simulink model "Trab_Tulior"  (R2020a)
settings: Solver=ode45  StartTime=0.0  StopTime=10  RelTol=1e-3  EnableMultiTasking=on
libraries: simulink x2
settings Model: Creator=20211en20246  LastModifiedBy=João Fernando Rangel
settings DataIOCC: LimitDataPoints=on  SaveFormat=Array  ReturnWorkspaceOutputs=off
settings OptimizationCC: LifeSpan=inf
settings DebuggingCC: UnderspecifiedInitializationDetection=Classic  MergeDetectMultiDrivingBlocksExec=none  SolverPrmCheckMsg=warning  SFUnexpectedBacktrackingDiag=warning  SFNoUnconditionalDefaultTransitionDiag=warning  SFExecutionAtInitializationDiag=none  ArithmeticOperatorsInVariantConditions=warning
settings HardwareCC: ProdBitPerPointer=32  ProdBitPerSizeT=32  ProdBitPerPtrDiffT=32  ProdLargestAtomicFloat=None  ProdIntDivRoundTo=Undefined  ProdEndianess=Unspecified  ProdWordSize=32  ProdHWDeviceType=32-bit Generic
settings ModelReferenceCC: PropagateSignalLabelsOutOfModel=off
settings SFSimCC: SimUseLocalCustomCode=off  CustomCodeUndefinedFunction=UseInterfaceOnly
settings RTWCC: RTWUseLocalCustomCode=off
settings CodeAppCC: StateflowObjectComments=on
settings GRTTargetCC: TargetLangStandard=C89/C90 (ANSI)
settings ConfigComp: CovMetricSettings=dw  CovHtmlReporting=on  CovSaveCumulativeToWorkspaceVar=on  CovSaveSingleToWorkspaceVar=on  CovExternalEMLEnable=off

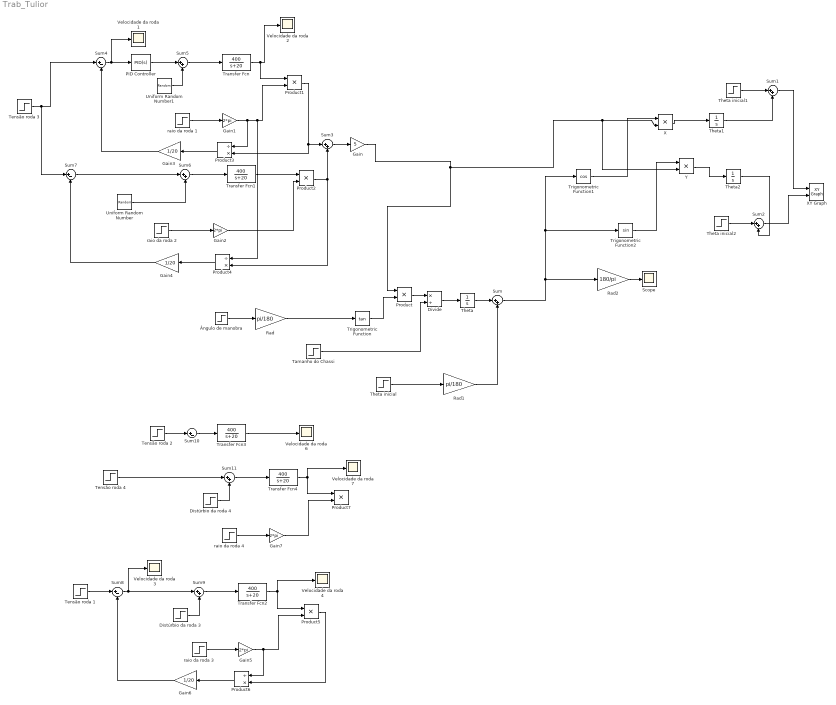
== system Trab_Tulior ==
  Distúrbio da roda 3 : Step  Time=0  After=0  SampleTime=0
  Distúrbio da roda 4 : Step  Time=0  After=0  SampleTime=0
  Divide : Product  Inputs=*/
  Gain : Gain  Gain=5
  Gain{1..2,5,7} (4 alike) : Gain  Gain=2*pi
  Gain3 : Gain  Gain=1/20
  Gain4 : Gain  Gain=1/20
  Gain6 : Gain  Gain=1/20
  PID Controller : simulink/Continuous/PID Controller  Controller=PID  Form=Parallel  TimeDomain=Continuous-time  UseExternalTs=off  SampleTime=-1  IntegratorMethod=Forward Euler  FilterMethod=Forward Euler  ControllerParametersSource=internal  P=77.31  I=171.77  D=1.28  UseFilter=on  N=100  TunerSelectOption=Transfer Function Based (PID Tuner App)  InitialConditionSource=internal  InitialConditionForIntegrator=0  InitialConditionForFilter=0  DifferentiatorICPrevScaledInput=0  ExternalReset=none  TrackingMode=off  Kt=1  LimitOutput=off  UpperSaturationLimit=inf  LowerSaturationLimit=-inf  LinearizeAsGain=on  AntiWindupMode=none  Kb=1  POutMin=[]  POutMax=[]  IOutMin=[]  IOutMax=[]  DOutMin=[]  DOutMax=[]  NOutMin=[]  NOutMax=[]  SumOutMin=[]  SumOutMax=[]  SaturationOutMin=[]  SaturationOutMax=[]  PParamMin=[]  PParamMax=[]  IParamMin=[]  IParamMax=[]  DParamMin=[]  DParamMax=[]  NParamMin=[]  NParamMax=[]  KbParamMin=[]  KbParamMax=[]  KtParamMin=[]  KtParamMax=[]  KbOutMin=[]  KbOutMax=[]  KtOutMin=[]  KtOutMax=[]  IntegratorOutMin=[]  IntegratorOutMax=[]  FilterOutMin=[]  FilterOutMax=[]  SumI1OutMin=[]  SumI1OutMax=[]  SumI2OutMin=[]  SumI2OutMax=[]  SumI3OutMin=[]  SumI3OutMax=[]  SumI4OutMin=[]  SumI4OutMax=[]  SumDOutMin=[]  SumDOutMax=[]  DifferentiatorOutMin=[]  DifferentiatorOutMax=[]  FilterDiffOutCoefMin=[]  FilterDiffOutCoefMax=[]  ReciprocalOutMin=[]  ReciprocalOutMax=[]  SumDenOutMin=[]  SumDenOutMax=[]  SumNumOutMin=[]  SumNumOutMax=[]  DivideOutMin=[]  DivideOutMax=[]  UdiffTsProdOutMin=[]  UdiffTsProdOutMax=[]  NTsProdOutMin=[]  NTsProdOutMax=[]  UintegralTsProdOutMin=[]  UintegralTsProdOutMax=[]  UngainTsProdOutMin=[]  UngainTsProdOutMax=[]  IntegratorContinuousStateAttributes=''  IntegratorStateMustResolveToSignalObject=off  IntegratorRTWStateStorageClass=Auto  FilterContinuousStateAttributes=''  FilterStateMustResolveToSignalObject=off  FilterRTWStateStorageClass=Auto  ParallelPVariant=InternalParameters  IdealPVariant=Disabled  IVariant=InternalParameters  DVariant=InternalParameters  IntegratorVariant=Continuous  SatVariant=Disabled  AWVariant=Passthrough  PCopyVariant=Disabled  TRVariant=Disabled  FdbkBlocksVariant=Forward  IdealPFdbkVariant=Disabled  SatFdbkVariant=Disabled  DerivativeFilterVariant=ContFilter  NVariant=InternalParameters  NCopyVariant=Disabled  FilterICVariant=InternalICsFilter  IntegratorICVariant=InternalICs  ExternalResetVariant=Disabled  TRSumVariant=Passthrough  SumFdbkVariant=Disabled  SumVariant=Sum_PID  TsampFilterVariant=InternalTs  TsampNgainVariant=Passthrough  TsampIntegralVariant=Passthrough
  Product{,1..2,5,7} (5 alike) : Product
  Product3 : Product  Inputs=/*
  Product4 : Product  Inputs=/*
  Product6 : Product  Inputs=/*
  Rad : Gain  Gain=pi/180
  Rad1 : Gain  Gain=pi/180
  Rad2 : Gain  Gain=180/pi
  Scope : Scope
  Sum{,1..3,5..6,9,11} (8 alike) : Sum  Inputs=|++
  Sum{4,7..8,10} (4 alike) : Sum  Inputs=|+-
  Tamanho do Chassi : Step  Time=0  After=0.44  SampleTime=0
  Tensão roda 1 : Step  Time=0  SampleTime=0
  Tensão roda 2 : Step  SampleTime=0
  Tensão roda 3 : Step  Time=0  SampleTime=0
  Tensão roda 4 : Step  Time=0  SampleTime=0
  Theta : Integrator
  Theta inicial : Step  Time=0  After=0  SampleTime=0
  Theta inicial1 : Step  Time=0  After=0  SampleTime=0
  Theta inicial2 : Step  Time=0  After=0  SampleTime=0
  Theta1 : Integrator
  Theta2 : Integrator
  Transfer Fcn{,1..4} (5 alike) : TransferFcn  Numerator=[400]  Denominator=[1 20]
  Trigonometric Function : Trigonometry  Operator=tan
  Trigonometric Function1 : Trigonometry  Operator=cos
  Trigonometric Function2 : Trigonometry
  Uniform Random Number : UniformRandomNumber  Minimum=-0.1  Maximum=5  SampleTime=0.1
  Uniform Random Number1 : UniformRandomNumber  Minimum=-0.1  Maximum=5  SampleTime=0.1
  Velocidade da roda {1..4,6..7} (6 alike) : Scope
  X : Product
  XY Graph : simulink/Sinks/XY Graph  xmin=-2  xmax=2  ymin=-2  ymax=2  st=-1
  Y : Product
  raio da roda {1..4} (4 alike) : Step  Time=0  After=0.080  SampleTime=0
  Ângulo de manobra : Step  Time=0  After=30  SampleTime=0
  wires:
  Gain/1 -> Y/2, X/2, Product/1
  Trigonometric Function/1 -> Product/2
  Tamanho do Chassi/1 -> Divide/2
  Divide/1 -> Theta/1
  Ângulo de manobra/1 -> Rad/1
  Rad/1 -> Trigonometric Function/1
  Rad2/1 -> Scope/1
  Trigonometric Function1/1 -> X/1
  Trigonometric Function2/1 -> Y/1
  X/1 -> Theta1/1
  Y/1 -> Theta2/1
  Sum/1 -> Trigonometric Function1/1, Trigonometric Function2/1, Rad2/1
  Theta inicial/1 -> Rad1/1
  Theta/1 -> Sum/1
  Rad1/1 -> Sum/2
  Product/1 -> Divide/1
  Theta inicial1/1 -> Sum1/1
  Theta1/1 -> Sum1/2
  Sum1/1 -> XY Graph/1
  Theta inicial2/1 -> Sum2/1
  Theta2/1 -> Sum2/2
  Sum2/1 -> XY Graph/2
  Transfer Fcn1/1 -> Product2/1
  Product2/1 -> Product4/2, Sum3/2
  Sum3/1 -> Gain/1
  Tensão roda 3/1 -> Sum4/1, Sum7/1
  Uniform Random Number1/1 -> Sum5/2
  Sum5/1 -> Transfer Fcn/1
  Sum6/1 -> Transfer Fcn1/1
  Uniform Random Number/1 -> Sum6/2
  Sum7/1 -> Sum6/1
  raio da roda 1/1 -> Gain1/1
  Gain1/1 -> Product3/1, Product4/1, Product1/2
  raio da roda 2/1 -> Gain2/1
  Gain2/1 -> Product2/2
  Product1/1 -> Product3/2, Sum3/1
  Sum4/1 -> PID Controller/1, Velocidade da roda 1/1
  Transfer Fcn/1 -> Product1/1, Velocidade da roda 2/1
  Product3/1 -> Gain3/1
  Product4/1 -> Gain4/1
  Gain4/1 -> Sum7/2
  Gain3/1 -> Sum4/2
  Product6/1 -> Gain6/1
  Transfer Fcn2/1 -> Product5/1, Velocidade da roda 4/1
  Gain5/1 -> Product6/1, Product5/2
  Sum8/1 -> Sum9/1, Velocidade da roda 3/1
  Distúrbio da roda 3/1 -> Sum9/2
  Product5/1 -> Product6/2
  raio da roda 3/1 -> Gain5/1
  Sum9/1 -> Transfer Fcn2/1
  Gain6/1 -> Sum8/2
  Tensão roda 1/1 -> Sum8/1
  Transfer Fcn3/1 -> Velocidade da roda 6/1
  Sum11/1 -> Transfer Fcn4/1
  Distúrbio da roda 4/1 -> Sum11/2
  Gain7/1 -> Product7/2
  Transfer Fcn4/1 -> Product7/1, Velocidade da roda 7/1
  Tensão roda 4/1 -> Sum11/1
  raio da roda 4/1 -> Gain7/1
  Tensão roda 2/1 -> Sum10/1
  Sum10/1 -> Transfer Fcn3/1
  PID Controller/1 -> Sum5/1
